simulink model "Quadcopter_Hinfinity_Discrete"  (R2016b)
settings: Solver=ode45  StartTime=0.0  StopTime=500  RelTol=1e-3  EnableMultiTasking=on
undefined symbols (not defined in the file or in its folder): A, B, C, D, g, K1d, m, Ts, X0
settings Model: Creator=Toshiba  LastModifiedBy=AAstudillo
settings DataIOCC: LimitDataPoints=on  SaveFormat=Array  SignalLoggingSaveFormat=ModelDataLogs
settings OptimizationCC: LifeSpan=inf
settings DebuggingCC: SolverPrmCheckMsg=warning  MultiTaskDSMMsg=warning  MultiTaskCondExecSysMsg=none  SFUnexpectedBacktrackingDiag=warning  SFNoUnconditionalDefaultTransitionDiag=warning  SFExecutionAtInitializationDiag=none
settings HardwareCC: ProdBitPerPointer=32  ProdBitPerSizeT=32  ProdBitPerPtrDiffT=32  ProdLargestAtomicFloat=None  ProdIntDivRoundTo=Undefined  ProdEndianess=Unspecified  ProdWordSize=32  ProdHWDeviceType=32-bit Generic
settings ModelReferenceCC: PropagateSignalLabelsOutOfModel=off
settings GRTTargetCC: TargetLangStandard=C89/C90 (ANSI)  GeneratePreprocessorConditionals=Disable all
settings ConfigComp: CovMetricSettings=dw  CovHtmlReporting=on  CovSaveCumulativeToWorkspaceVar=on  CovSaveSingleToWorkspaceVar=on  CovExternalEMLEnable=off

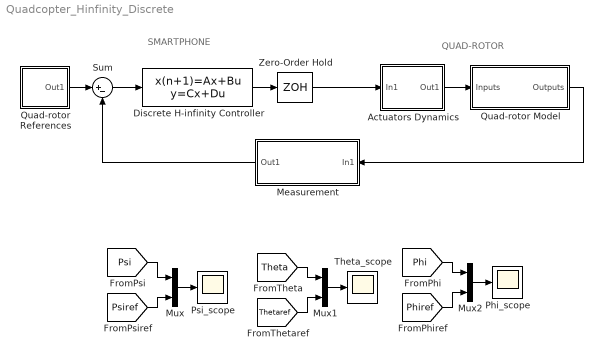
== system Quadcopter_Hinfinity_Discrete ==
  note: QUAD-ROTOR
  note: SMARTPHONE
  Actuators Dynamics : Subsystem
  Discrete H-infinity Controller : DiscreteStateSpace  A=K1d.A  B=K1d.B  C=K1d.C  D=K1d.D  X0=zeros(size(K1d.A,1),1)  SampleTime=Ts
  Measurement : Subsystem
  Mux : Mux  Inputs=2
  Mux1 : Mux  Inputs=2
  Mux2 : Mux  Inputs=2
  Phi_scope : Scope
  Psi_scope : Scope
  Quad-rotor Model : Subsystem
  Quad-rotor References : Subsystem
  Sum : Sum  Inputs=|+-
  Theta_scope : Scope
  Zero-Order Hold : ZeroOrderHold  SampleTime=Ts
  wires:
  Quad-rotor References/1(Out1) -> Sum/1
  Mux/1 -> Psi_scope/1
  Mux1/1 -> Theta_scope/1
  Mux2/1 -> Phi_scope/1
  [Psi] -> Mux/1
  [Psiref] -> Mux/2
  [Theta] -> Mux1/1
  [Thetaref] -> Mux1/2
  [Phi] -> Mux2/1
  [Phiref] -> Mux2/2
  Sum/1 -> Discrete H-infinity Controller/1
  Discrete H-infinity Controller/1 -> Zero-Order Hold/1
  Measurement/1(Out1) -> Sum/2
  Quad-rotor Model/1(Outputs) -> Measurement/1(In1)
  Actuators Dynamics/1(Out1) -> Quad-rotor Model/1(Inputs)
  Zero-Order Hold/1 -> Actuators Dynamics/1(In1)

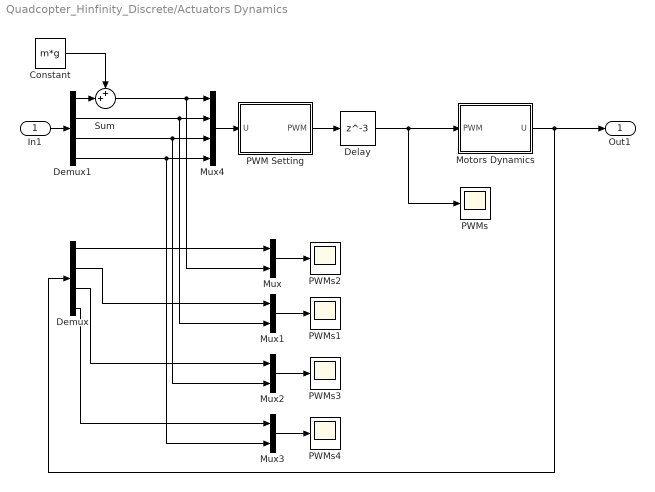
== system Quadcopter_Hinfinity_Discrete/Actuators Dynamics ==
  In1 : Inport
  Constant : Constant  Value=m*g  VectorParams1D=off
  Delay : Delay  DelayLength=3  SampleTime=Ts
  Demux : Demux
  Demux1 : Demux
  Motors Dynamics : MATLAB Function  TreatAsAtomicUnit=on
  Mux{,1..3} (4 alike) : Mux  Inputs=2
  Mux4 : Mux
  PWM Setting : MATLAB Function  TreatAsAtomicUnit=on
  PWMs{,1..4} (5 alike) : Scope
  Sum : Sum  Inputs=++|
  Out1 : Outport
  wires:
  In1/1 -> Demux1/1
  Motors Dynamics/1(U) -> Demux/1, Out1/1
  Mux/1 -> PWMs2/1
  Mux1/1 -> PWMs1/1
  Mux2/1 -> PWMs3/1
  Mux3/1 -> PWMs4/1
  Demux/1 -> Mux/1
  Demux/2 -> Mux1/1
  Demux/3 -> Mux2/1
  Demux/4 -> Mux3/1
  Constant/1 -> Sum/1
  Demux1/1 -> Sum/2
  Sum/1 -> Mux/2, Mux4/1
  Demux1/2 -> Mux1/2, Mux4/2
  Demux1/3 -> Mux2/2, Mux4/3
  Demux1/4 -> Mux3/2, Mux4/4
  Mux4/1 -> PWM Setting/1(U)
  PWM Setting/1(PWM) -> Delay/1
  Delay/1 -> PWMs/1, Motors Dynamics/1(PWM)

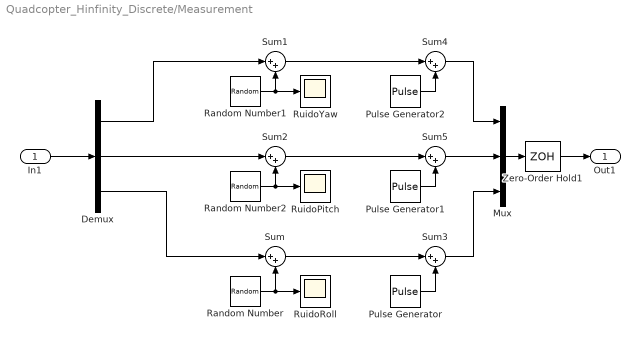
== system Quadcopter_Hinfinity_Discrete/Measurement ==
  In1 : Inport
  Demux : Demux  Outputs=3
  Mux : Mux  Inputs=3
  Pulse Generator : DiscretePulseGenerator  PulseType=Time based  Amplitude=0.2  Period=15  PulseWidth=2  PhaseDelay=5
  Pulse Generator1 : DiscretePulseGenerator  PulseType=Time based  Amplitude=0.2  Period=15  PulseWidth=2
  Pulse Generator2 : DiscretePulseGenerator  PulseType=Time based  Amplitude=0.2  Period=15  PhaseDelay=10
  Random Number : RandomNumber  Variance=0.005  SampleTime=Ts
  Random Number1 : RandomNumber  Variance=0.0005  SampleTime=Ts
  Random Number2 : RandomNumber  Variance=0.005  SampleTime=Ts
  RuidoPitch : Scope
  RuidoRoll : Scope
  RuidoYaw : Scope
  Sum{,1..5} (6 alike) : Sum  Inputs=|++
  Zero-Order Hold1 : ZeroOrderHold  SampleTime=Ts
  Out1 : Outport
  wires:
  Zero-Order Hold1/1 -> Out1/1
  Mux/1 -> Zero-Order Hold1/1
  Random Number/1 -> Sum/2, RuidoRoll/1
  Demux/3 -> Sum/1
  Demux/1 -> Sum1/1
  Random Number2/1 -> RuidoPitch/1, Sum2/2
  Demux/2 -> Sum2/1
  Random Number1/1 -> RuidoYaw/1, Sum1/2
  In1/1 -> Demux/1
  Pulse Generator/1 -> Sum3/2
  Pulse Generator1/1 -> Sum5/2
  Pulse Generator2/1 -> Sum4/2
  Sum2/1 -> Sum5/1
  Sum1/1 -> Sum4/1
  Sum/1 -> Sum3/1
  Sum4/1 -> Mux/1
  Sum5/1 -> Mux/2
  Sum3/1 -> Mux/3

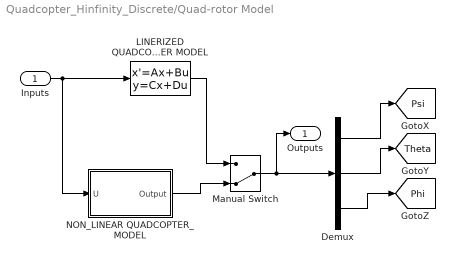
== system Quadcopter_Hinfinity_Discrete/Quad-rotor Model ==
  Inputs : Inport
  Demux : Demux  Outputs=3
  LINERIZED QUADCOPTER MODEL : StateSpace  A=A  B=B  C=C  D=D  X0=X0
  Manual Switch : ManualSwitch  CurrentSetting=0
  NON_LINEAR QUADCOPTER_MODEL : Subsystem
  Outputs : Outport
  tag scope: Phi=global, Psi=global, Theta=global
  wires:
  Inputs/1 -> LINERIZED QUADCOPTER MODEL/1, NON_LINEAR QUADCOPTER_MODEL/1(U)
  LINERIZED QUADCOPTER MODEL/1 -> Manual Switch/1
  Manual Switch/1 -> Outputs/1, Demux/1
  NON_LINEAR QUADCOPTER_MODEL/1("Output ") -> Manual Switch/2
  Demux/3 -> [Phi]
  Demux/2 -> [Theta]
  Demux/1 -> [Psi]

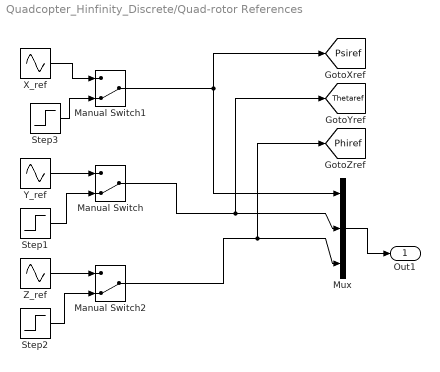
== system Quadcopter_Hinfinity_Discrete/Quad-rotor References ==
  Manual Switch : ManualSwitch  CurrentSetting=0
  Manual Switch1 : ManualSwitch  CurrentSetting=0
  Manual Switch2 : ManualSwitch  CurrentSetting=0
  Mux : Mux  Inputs=3
  Step1 : Step  Time=15  After=0  SampleTime=Ts
  Step2 : Step  Time=10  After=0  SampleTime=Ts
  Step3 : Step  Time=5  After=0  SampleTime=Ts
  X_ref : Sin  Frequency=3.141592654*0.1  SampleTime=0
  Y_ref : Sin  Frequency=3.141592654*0.1  Phase=3.141592654/2  SampleTime=0
  Z_ref : Sin  Bias=1  Frequency=3.141592654*0.05  Phase=3.141592654  SampleTime=0
  Out1 : Outport
  tag scope: Phiref=global, Psiref=global, Thetaref=global
  wires:
  Mux/1 -> Out1/1
  X_ref/1 -> Manual Switch1/1
  Manual Switch1/1 -> [Psiref], Mux/1
  Step3/1 -> Manual Switch1/2
  Y_ref/1 -> Manual Switch/1
  Step1/1 -> Manual Switch/2
  Manual Switch/1 -> [Thetaref], Mux/2
  Step2/1 -> Manual Switch2/2
  Z_ref/1 -> Manual Switch2/1
  Manual Switch2/1 -> [Phiref], Mux/3

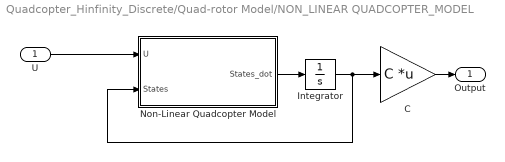
== system Quadcopter_Hinfinity_Discrete/Quad-rotor Model/NON_LINEAR QUADCOPTER_MODEL ==
  U : Inport
  C : Gain  Gain=C  Multiplication=Matrix(K*u)
  Integrator : Integrator  InitialCondition=X0
  Non-Linear Quadcopter Model : MATLAB Function  TreatAsAtomicUnit=on
  "Output " : Outport
  wires:
  Non-Linear Quadcopter Model/1(States_dot) -> Integrator/1
  Integrator/1 -> Non-Linear Quadcopter Model/2(States), C/1
  U/1 -> Non-Linear Quadcopter Model/1(U)
  C/1 -> "Output "/1

== matlab function Quadcopter_Hinfinity_Discrete/Actuators Dynamics/PWM Setting ==
  data: U input; PWM output
function PWM = fcn(U)

M_inv = [0.2500   11.9048   -1.4490   -1.4490;
        0.2500  -11.9048   -1.4490    1.4490;
        0.2500   11.9048    1.4490    1.4490;
        0.2500  -11.9048    1.4490   -1.4490];

Force = M_inv*U;

% if Force(1) < 0
%     Force(3) = Force(3) - Force(1);
% end
% if Force(2) < 0
%     Force(4) = Force(4) - Force(2);
% end
% if Force(3) < 0
%     Force(1) = Force(1) - Force(3);
% end
% if Force(4) < 0
%     Force(2) = Force(2) - Force(4);
% end

PWM_1 =  -1.983*(Force(1)^2) + 47.84*Force(1) + 3.835; % PWM [0...255]
PWM_2 =  -1.983*(Force(2)^2) + 47.84*Force(2) + 3.835; % PWM [0...255]
PWM_3 =  -1.983*(Force(3)^2) + 47.84*Force(3) + 3.835; % PWM [0...255]
PWM_4 =  -1.983*(Force(4)^2) + 47.84*Force(4) + 3.835; % PWM [0...255]

if PWM_1 < 0
    PWM_3 = PWM_3 - PWM_1;
end
if PWM_2 < 0
    PWM_4 = PWM_4  - PWM_2;
end
if PWM_3 < 0
    PWM_1 = PWM_1 - PWM_3;
end
if Force(4) < 0
    PWM_2 = PWM_2 - PWM_4 ;
end

PWM_1 = min(255, max(0, PWM_1));
PWM_2 = min(255, max(0, PWM_2));
PWM_3 = min(255, max(0, PWM_3));
PWM_4 = min(255, max(0, PWM_4));

PWM = [PWM_1 PWM_2 PWM_3 PWM_4];

== matlab function Quadcopter_Hinfinity_Discrete/Quad-rotor Model/NON_LINEAR QUADCOPTER_MODEL/Non-Linear Quadcopter Model ==
  data: U input; States input; States_dot output
function States_dot  = fcn(U, States)

% Gravity constant
              g = 9.807;

              m = 1.568;
              Ixx = 0.0135;
              Iyy = 0.0124;
              Izz = 0.0336;

    %Inputs = U, States
    %Outputs = States_dot  
    %States: X dX Y dY Z dZ Psi dPsi Theta dTheta Phi dPhi
    %        1  2 3  4 5  6  7   8     9      10   11  12
    
    U1 = U(1);
    U2 = U(2);
    U3 = U(3);
    U4 = U(4);

    dPsi = States(2);
    ddPsi = (((Ixx-Iyy)/Izz)*States(6)*States(4)) + (U2/Izz);
    dTheta = States(4);
    ddTheta = (((Izz-Ixx)/Iyy)*States(6)*States(2)) + (U3/Iyy);
    dPhi = States(6);
    ddPhi = (((Iyy-Izz)/Ixx)*States(4)*States(2)) + (U4/Ixx);

    States_dot = [dPsi, ddPsi, dTheta, ddTheta, dPhi, ddPhi]';

== matlab function Quadcopter_Hinfinity_Discrete/Actuators Dynamics/Motors Dynamics ==
  data: PWM input; U output
function U = fcn(PWM)

F_M1 = (5.441e-5)*(PWM(1)^2) + 0.01586*PWM(1) + 0.014808;
F_M2 = (5.441e-5)*(PWM(2)^2) + 0.01586*PWM(2) + 0.014808;
F_M3 = (5.441e-5)*(PWM(3)^2) + 0.01586*PWM(3) + 0.014808;
F_M4 = (5.441e-5)*(PWM(4)^2) + 0.01586*PWM(4) + 0.014808;

Force = [F_M1 F_M2 F_M3 F_M4]';

M = [1.0000    1.0000    1.0000    1.0000;
    0.0210   -0.0210    0.0210   -0.0210;
   -0.1725   -0.1725    0.1725    0.1725;
   -0.1725    0.1725    0.1725   -0.1725];

g = 9.807;
m = 1.568;

U = M*Force;
